simulink model "PropTest"  (R2019b)
settings: Solver=VariableStepAuto  StartTime=0.0  StopTime=40  RelTol=1e-3
values from neighbouring files (symbols this model uses):
  BackProp =     [back_prop.mat]
  ForwProp =     [forward_prop.mat]
undefined symbols (not defined in the file or in its folder): DiscIntNeverNeededParam, motor
libraries: fl_lib x27, nesl_utility x12, sharedutil x3, fl_ps_legacy_lib x3, ee_lib x3, sdl_lib x3, simulink x2
(part 1 of 2)
settings Model: Creator=gonza  LastModifiedBy=gonza

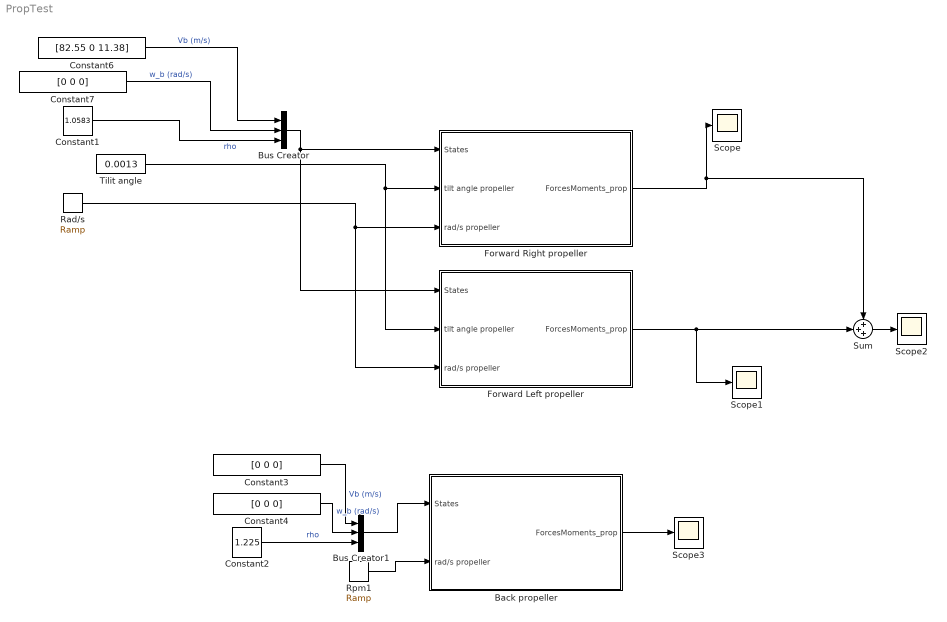
== system PropTest ==
  Back propeller : Subsystem
  Bus Creator : BusCreator  Inputs=3
  Bus Creator1 : BusCreator  Inputs=3
  Constant1 : Constant  Value=1.0583
  Constant2 : Constant  Value=1.225
  Constant3 : Constant  Value=[0 0 0]
  Constant4 : Constant  Value=[0 0 0]
  Constant6 : Constant  Value=[82.55 0 11.38]
  Constant7 : Constant  Value=[0 0 0]
  Forward Left propeller : Subsystem
  Forward Right propeller : Subsystem
  Rad/s : simulink/Sources/Ramp  slope=5  start=5  InitialOutput=10
  Rpm1 : simulink/Sources/Ramp  slope=25  start=5  InitialOutput=0
  Scope{,1..3} (4 alike) : Scope
  Sum : Sum  Inputs=+++
  "Tilit angle " : Constant  Value=0.0013
  wires:
  Bus Creator/1 -> Forward Right propeller/1(States), Forward Left propeller/1(States)
  Constant4/1 -> Bus Creator1/2  "w_b (rad/s)"
  Bus Creator1/1 -> Back propeller/1(States)
  Forward Left propeller/1(ForcesMoments_prop) -> Scope1/1, Sum/2
  Constant1/1 -> Bus Creator/3  "rho"
  Rad/s/1 -> Forward Right propeller/3(rad/s propeller), Forward Left propeller/3(rad/s propeller)
  Forward Right propeller/1(ForcesMoments_prop) -> Scope/1, Sum/1
  Sum/1 -> Scope2/1
  "Tilit angle "/1 -> Forward Right propeller/2(tilt angle propeller), Forward Left propeller/2(tilt angle propeller)
  Constant7/1 -> Bus Creator/2  "w_b (rad/s)"
  Constant2/1 -> Bus Creator1/3  "rho"
  Constant6/1 -> Bus Creator/1  "Vb (m/s)"
  Rpm1/1 -> Back propeller/2(rad/s propeller)
  Constant3/1 -> Bus Creator1/1  "Vb (m/s)"
  Back propeller/1(ForcesMoments_prop) -> Scope3/1

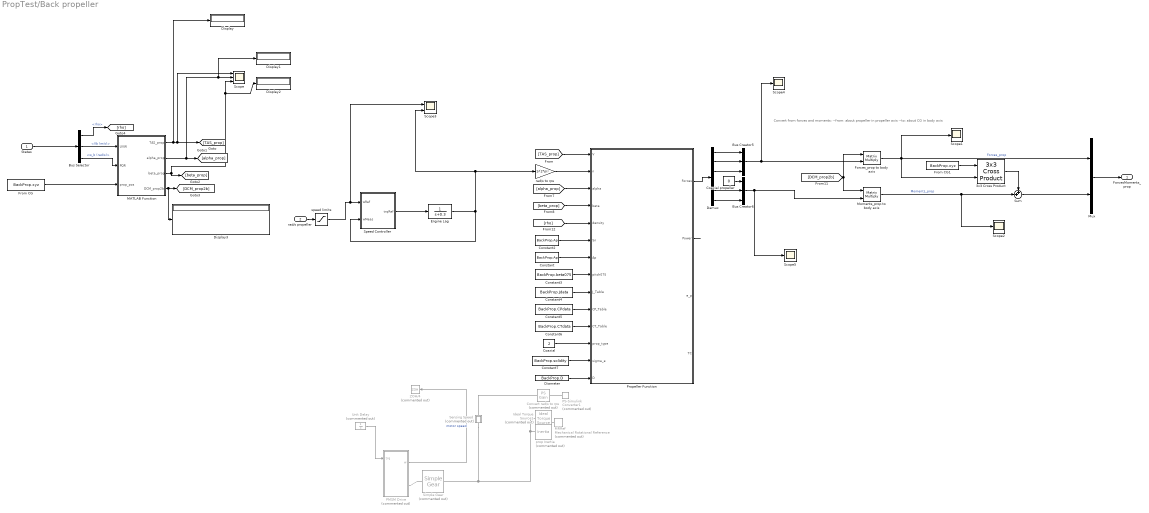
== system PropTest/Back propeller ==
  note: Convert from forces and moments: --from: about propeller in propeller axis --to: about CG in body axis
  States : Inport
  rad/s propeller : Inport  Port=2
  3x3 Cross Product : sharedutil/3x3 Cross Product  aMode=aMode
      settings: SourceProductBaseCode=AE
  Bus Creator5 : BusCreator  Inputs=3
  Bus Creator6 : BusCreator  Inputs=3
  Bus Selector : BusSelector  OutputSignals=rho,Vb (m/s),w_b (rad/s)
  "Coaxial " : Constant  Value=2
  Coaxial propeller : Constant  Value=0
  Constant : Constant  Value=BackProp.Ap
  Constant2 : Constant  Value=BackProp.Ap
  Constant3 : Constant  Value=BackProp.beta075
  Constant4 : Constant  Value=BackProp.Jdata
  Constant5 : Constant  Value=BackProp.CPdata
  Constant6 : Constant  Value=BackProp.CTdata
  Constant7 : Constant  Value=BackProp.solidity
  Convert rad/s to rps : fl_ps_legacy_lib/Legacy Physical Signals/Functions/PS Gain  Commented=on  gain=1/(2*pi)
      settings: SourceProductName=Simscape
  Demux : Demux  Outputs=6
  Diameter : Constant  Value=BackProp.D
  Display{,1..3} (4 alike) : Display
  Engine Lag : TransferFcn  Denominator=[1 0.3]  ContinuousStateAttributes='EngineLag'
  Forces_prop to body axis : Product  Multiplication=Matrix(*)
  From CG : Constant  Value=BackProp.xyz
  From CG1 : Constant  Value=BackProp.xyz
  Ideal Torque Source1 : fl_lib/Mechanical/Mechanical Sources/Ideal Torque Source  Commented=on
  MATLAB Function : MATLAB Function  TreatAsAtomicUnit=on
  MRRef : fl_lib/Mechanical/Rotational Elements/Mechanical Rotational Reference  Commented=on
  Moments_prop to body axis : Product  Multiplication=Matrix(*)
  Mux : Mux  Inputs=2
  PMSM Drive : Subsystem  Tag=PublishSubsystem  Commented=on  VariantControl=Variant1
  PS-Simulink Converter1 : nesl_utility/PS-Simulink Converter  Commented=on  PhysicalDomain=network_engine_domain  SubClassName=ps_output  LeftPortType=input  RightPortType=output  PseudoPeriodic=off  Frequencies=[]  Unit=inherit  AffineConversion=off
  Propeller Function : MATLAB Function  TreatAsAtomicUnit=on
  Scope : Scope  NumInputPorts=3
  Scope{1..2,4..5} (4 alike) : Scope
  Scope3 : Scope  NumInputPorts=2
  Sensing Speed : Subsystem  Commented=on
      mask Display: disp('w')
  Simple Gear : sdl_lib/Gears/Simple Gear  Commented=on  ratio=motor.gear_reduction_forward  rotation_direction=1  friction_model=sdl.enum.gear_efficiencies_load.off  T_noload=0.1 N*m  T_nom=5 N*m  efficiency_nom=0.8  efficiency=0.8  mu_visc=[0, 0] N*m/(rad/s)  w_thr=0.01 rad/s  pwr_thr=0.001 W  enable_faults=simscape.enum.onoff.off  efficiency_fault=0.05  external_fault=simscape.enum.onoff.off  temporal_fault=simscape.enum.onoff.off  fault_time=5 s  fault_angles=pi / 12 rad  report_fault=1  temperature_TLU=[280, 300, 320] K  load_TLU=[1, 5, 10] N*m  efficiency_TLU=[.95, .9, .85]  efficiency_TLU2=[.85, .8, .75; .95, .9, .85; .85, .8, .7]  thermal_mass=50 J/K  T_init=300 K
      settings: SourceProductName=Simscape Driveline
  Speed Controller : Subsystem  mask(P+I motor speed controller){Kp=10, Ki=1, trqMax=20000, ts=0.01}
      mask prompts: Kp "Proportional gain (Nm/(rad/s))"; Ki "Integral gain (Nm/rad)"; trqMax "Maximum torque demand"; ts "Sample time"
      mask help: Inputs wRef and wMeas are the demanded rotor speed and measured rotor speed in rad/s. The controller output is a torque demand in Nm.
  Sum : Sum  Inputs=++|
  Unit Delay : UnitDelay  Commented=on  SampleTime=0.01  HasFrameUpgradeWarning=on
  ZOH/4 : ZeroOrderHold  Commented=on  SampleTime=0.01
  prop Inertia : fl_lib/Mechanical/Rotational Elements/Inertia  Commented=on  inertia="ForwProp.inertia  kg*m^2"  w_specify=on  w_priority=High  w=0 rpm  w_nominal_specify=off  w_nominal_unit=rad/s  w_nominal_value=1  t_specify=off  t_priority=High  t=0 N*m  t_nominal_specify=off  t_nominal_unit=N*m  t_nominal_value=1
  rad/s to rps : Gain  Gain=1/(2*pi)
  speed limits : Saturate  UpperLimit=2000  LowerLimit=-1500
  ForcesMoments_prop : Outport
  wires:
  [rho] -> Propeller Function/5(density)
  MATLAB Function/2(alpha_prop) -> [alpha_prop], Display1/1, Scope/2
  MATLAB Function/3(beta_prop) -> [beta_prop], Scope/3, Display2/1
  Unit Delay/1 -> PMSM Drive/1(trq)
  MATLAB Function/1(TAS_prop) -> Display/1, [TAS_prop], Scope/1
  MATLAB Function/4(DCM_prop2b) -> Display3/1, [DCM_prop2b]
  [TAS_prop] -> Propeller Function/1(V)
  PMSM Drive/1(w) -> ZOH/4/1  "motor speed"
  speed limits/1 -> Scope3/1, Speed Controller/1(wRef)
  From CG/1 -> MATLAB Function/3(prop_pos)
  [alpha_prop] -> Propeller Function/3(alpha)
  rad/s propeller/1 -> speed limits/1
  States/1 -> Bus Selector/1
  Bus Selector/2 -> MATLAB Function/1(UVW)  "<Vb (m/s)>"
  Bus Selector/3 -> MATLAB Function/2(PQR)  "<w_b (rad/s)>"
  Bus Selector/1 -> [rho]  "<rho>"
  Mux/1 -> ForcesMoments_prop/1
  3x3 Cross Product/1 -> Sum/1
  Moments_prop to body axis/1 -> Scope2/1, Sum/2  "Moments_prop"
  Forces_prop to body axis/1 -> Scope1/1, 3x3 Cross Product/2, Mux/1  "Forces_prop"
  [DCM_prop2b] -> Forces_prop to body axis/1, Moments_prop to body axis/1
  From CG1/1 -> 3x3 Cross Product/1
  Bus Creator6/1 -> Scope5/1, Moments_prop to body axis/2
  Sum/1 -> Mux/2
  [beta_prop] -> Propeller Function/4(beta)
  Constant/1 -> Propeller Function/7(Ap)
  Constant2/1 -> Propeller Function/6(Sn)
  Constant3/1 -> Propeller Function/8(pitch075)
  Constant4/1 -> Propeller Function/9(J_Table)
  Constant5/1 -> Propeller Function/10(CP_Table)
  Constant6/1 -> Propeller Function/11(CT_Table)
  Constant7/1 -> Propeller Function/13(sigma_e)
  "Coaxial "/1 -> Propeller Function/12(prop_type)
  Propeller Function/1(Forces) -> Demux/1
  Demux/1 -> Bus Creator5/1
  Demux/6 -> Bus Creator6/3
  Demux/2 -> Bus Creator5/2
  Demux/3 -> Bus Creator5/3
  Demux/5 -> Bus Creator6/2
  Propeller Function/2(Power) -> ?
  Speed Controller/1(trqRef) -> Engine Lag/1
  Engine Lag/1 -> Speed Controller/2(wMeas), Scope3/2, rad/s to rps/1
  Diameter/1 -> Propeller Function/14(D)
  rad/s to rps/1 -> Propeller Function/2(n)
  Coaxial propeller/1 -> Bus Creator6/1
  Bus Creator5/1 -> Scope4/1, Forces_prop to body axis/2
  connections:
  Sensing Speed/LConn1 -- Simple Gear/RConn1 -- prop Inertia/LConn1 -- Ideal Torque Source1/LConn1
  Ideal Torque Source1/RConn2 -- MRRef/LConn1
  Sensing Speed/RConn1 -- Convert rad/s to rps/LConn1
  PS-Simulink Converter1/LConn1 -- Convert rad/s to rps/RConn1
  Simple Gear/LConn1 -- PMSM Drive/RConn1

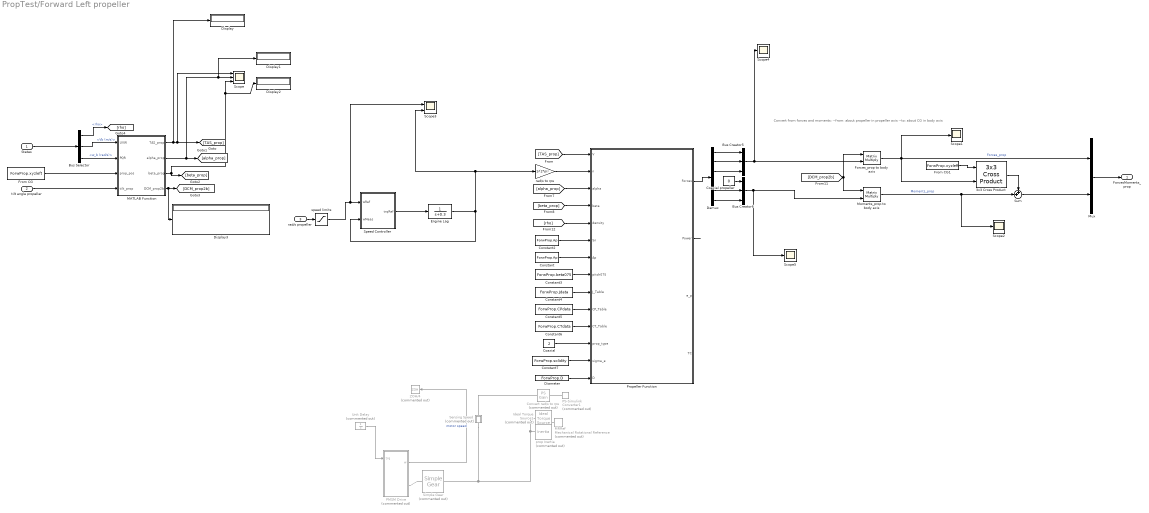
== system PropTest/Forward Left propeller ==
  note: Convert from forces and moments: --from: about propeller in propeller axis --to: about CG in body axis
  States : Inport
  tilt angle propeller : Inport  Port=2
  rad/s propeller : Inport  Port=3
  3x3 Cross Product : sharedutil/3x3 Cross Product  aMode=aMode
      settings: SourceProductBaseCode=AE
  Bus Creator5 : BusCreator  Inputs=3
  Bus Creator6 : BusCreator  Inputs=3
  Bus Selector : BusSelector  OutputSignals=rho,Vb (m/s),w_b (rad/s)
  "Coaxial " : Constant  Value=2
  Coaxial propeller : Constant  Value=0
  Constant : Constant  Value=ForwProp.Ap
  Constant2 : Constant  Value=ForwProp.Ap
  Constant3 : Constant  Value=ForwProp.beta075
  Constant4 : Constant  Value=ForwProp.Jdata
  Constant5 : Constant  Value=ForwProp.CPdata
  Constant6 : Constant  Value=ForwProp.CTdata
  Constant7 : Constant  Value=ForwProp.solidity
  Convert rad/s to rps : fl_ps_legacy_lib/Legacy Physical Signals/Functions/PS Gain  Commented=on  gain=1/(2*pi)
      settings: SourceProductName=Simscape
  Demux : Demux  Outputs=6
  Diameter : Constant  Value=ForwProp.D
  Display{,1..3} (4 alike) : Display
  Engine Lag : TransferFcn  Denominator=[1 0.3]  ContinuousStateAttributes='EngineLag'
  Forces_prop to body axis : Product  Multiplication=Matrix(*)
  From CG : Constant  Value=ForwProp.xyzleft
  From CG1 : Constant  Value=ForwProp.xyzleft
  Ideal Torque Source1 : fl_lib/Mechanical/Mechanical Sources/Ideal Torque Source  Commented=on
  MATLAB Function : MATLAB Function  TreatAsAtomicUnit=on
  MRRef : fl_lib/Mechanical/Rotational Elements/Mechanical Rotational Reference  Commented=on
  Moments_prop to body axis : Product  Multiplication=Matrix(*)
  Mux : Mux  Inputs=2
  PMSM Drive : Subsystem  Tag=PublishSubsystem  Commented=on  VariantControl=Variant1
  PS-Simulink Converter1 : nesl_utility/PS-Simulink Converter  Commented=on  PhysicalDomain=network_engine_domain  SubClassName=ps_output  LeftPortType=input  RightPortType=output  PseudoPeriodic=off  Frequencies=[]  Unit=inherit  AffineConversion=off
  Propeller Function : MATLAB Function  TreatAsAtomicUnit=on
  Scope : Scope  NumInputPorts=3
  Scope{1..2,4..5} (4 alike) : Scope
  Scope3 : Scope  NumInputPorts=2
  Sensing Speed : Subsystem  Commented=on
      mask Display: disp('w')
  Simple Gear : sdl_lib/Gears/Simple Gear  Commented=on  ratio=motor.gear_reduction_forward  rotation_direction=1  friction_model=sdl.enum.gear_efficiencies_load.off  T_noload=0.1 N*m  T_nom=5 N*m  efficiency_nom=0.8  efficiency=0.8  mu_visc=[0, 0] N*m/(rad/s)  w_thr=0.01 rad/s  pwr_thr=0.001 W  enable_faults=simscape.enum.onoff.off  efficiency_fault=0.05  external_fault=simscape.enum.onoff.off  temporal_fault=simscape.enum.onoff.off  fault_time=5 s  fault_angles=pi / 12 rad  report_fault=1  temperature_TLU=[280, 300, 320] K  load_TLU=[1, 5, 10] N*m  efficiency_TLU=[.95, .9, .85]  efficiency_TLU2=[.85, .8, .75; .95, .9, .85; .85, .8, .7]  thermal_mass=50 J/K  T_init=300 K
      settings: SourceProductName=Simscape Driveline
  Speed Controller : Subsystem  mask(P+I motor speed controller){Kp=10, Ki=1, trqMax=20000, ts=0.01}
      mask prompts: Kp "Proportional gain (Nm/(rad/s))"; Ki "Integral gain (Nm/rad)"; trqMax "Maximum torque demand"; ts "Sample time"
      mask help: Inputs wRef and wMeas are the demanded rotor speed and measured rotor speed in rad/s. The controller output is a torque demand in Nm.
  Sum : Sum  Inputs=++|
  Unit Delay : UnitDelay  Commented=on  SampleTime=0.01  HasFrameUpgradeWarning=on
  ZOH/4 : ZeroOrderHold  Commented=on  SampleTime=0.01
  prop Inertia : fl_lib/Mechanical/Rotational Elements/Inertia  Commented=on  inertia="ForwProp.inertia  kg*m^2"  w_specify=on  w_priority=High  w=0 rpm  w_nominal_specify=off  w_nominal_unit=rad/s  w_nominal_value=1  t_specify=off  t_priority=High  t=0 N*m  t_nominal_specify=off  t_nominal_unit=N*m  t_nominal_value=1
  rad/s to rps : Gain  Gain=1/(2*pi)
  speed limits : Saturate  UpperLimit=2000  LowerLimit=-1500
  ForcesMoments_prop : Outport
  wires:
  [rho] -> Propeller Function/5(density)
  MATLAB Function/2(alpha_prop) -> [alpha_prop], Display1/1, Scope/2
  MATLAB Function/3(beta_prop) -> [beta_prop], Scope/3, Display2/1
  Unit Delay/1 -> PMSM Drive/1(trq)
  MATLAB Function/1(TAS_prop) -> Display/1, [TAS_prop], Scope/1
  MATLAB Function/4(DCM_prop2b) -> Display3/1, [DCM_prop2b]
  tilt angle propeller/1 -> MATLAB Function/4(tilt_prop)
  [TAS_prop] -> Propeller Function/1(V)
  PMSM Drive/1(w) -> ZOH/4/1  "motor speed"
  speed limits/1 -> Scope3/1, Speed Controller/1(wRef)
  From CG/1 -> MATLAB Function/3(prop_pos)
  [alpha_prop] -> Propeller Function/3(alpha)
  rad/s propeller/1 -> speed limits/1
  States/1 -> Bus Selector/1
  Bus Selector/2 -> MATLAB Function/1(UVW)  "<Vb (m/s)>"
  Bus Selector/3 -> MATLAB Function/2(PQR)  "<w_b (rad/s)>"
  Bus Selector/1 -> [rho]  "<rho>"
  Mux/1 -> ForcesMoments_prop/1
  3x3 Cross Product/1 -> Sum/1
  Moments_prop to body axis/1 -> Scope2/1, Sum/2  "Moments_prop"
  Forces_prop to body axis/1 -> Scope1/1, 3x3 Cross Product/2, Mux/1  "Forces_prop"
  [DCM_prop2b] -> Forces_prop to body axis/1, Moments_prop to body axis/1
  From CG1/1 -> 3x3 Cross Product/1
  Bus Creator6/1 -> Scope5/1, Moments_prop to body axis/2
  Bus Creator5/1 -> Scope4/1, Forces_prop to body axis/2
  Sum/1 -> Mux/2
  [beta_prop] -> Propeller Function/4(beta)
  Constant/1 -> Propeller Function/7(Ap)
  Constant2/1 -> Propeller Function/6(Sn)
  Constant3/1 -> Propeller Function/8(pitch075)
  Constant4/1 -> Propeller Function/9(J_Table)
  Constant5/1 -> Propeller Function/10(CP_Table)
  Constant6/1 -> Propeller Function/11(CT_Table)
  Constant7/1 -> Propeller Function/13(sigma_e)
  "Coaxial "/1 -> Propeller Function/12(prop_type)
  Propeller Function/1(Forces) -> Demux/1
  Demux/1 -> Bus Creator5/1
  Demux/6 -> Bus Creator6/3
  Demux/2 -> Bus Creator5/2
  Demux/3 -> Bus Creator5/3
  Demux/5 -> Bus Creator6/2
  Propeller Function/2(Power) -> ?
  Speed Controller/1(trqRef) -> Engine Lag/1
  Engine Lag/1 -> Speed Controller/2(wMeas), Scope3/2, rad/s to rps/1
  Diameter/1 -> Propeller Function/14(D)
  rad/s to rps/1 -> Propeller Function/2(n)
  Coaxial propeller/1 -> Bus Creator6/1
  connections:
  Sensing Speed/LConn1 -- Simple Gear/RConn1 -- prop Inertia/LConn1 -- Ideal Torque Source1/LConn1
  Ideal Torque Source1/RConn2 -- MRRef/LConn1
  Sensing Speed/RConn1 -- Convert rad/s to rps/LConn1
  PS-Simulink Converter1/LConn1 -- Convert rad/s to rps/RConn1
  Simple Gear/LConn1 -- PMSM Drive/RConn1

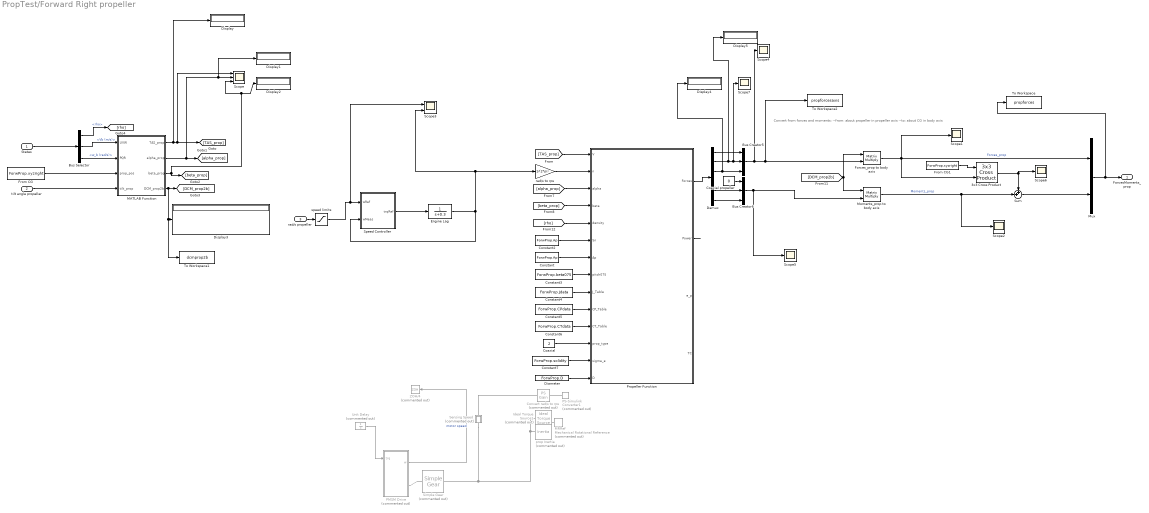
== system PropTest/Forward Right propeller ==
  note: Convert from forces and moments: --from: about propeller in propeller axis --to: about CG in body axis
  States : Inport
  tilt angle propeller : Inport  Port=2
  rad/s propeller : Inport  Port=3
  3x3 Cross Product : sharedutil/3x3 Cross Product  aMode=aMode
      settings: SourceProductBaseCode=AE
  Bus Creator5 : BusCreator  Inputs=3
  Bus Creator6 : BusCreator  Inputs=3
  Bus Selector : BusSelector  OutputSignals=rho,Vb (m/s),w_b (rad/s)
  "Coaxial " : Constant  Value=2
  Coaxial propeller : Constant  Value=0
  Constant : Constant  Value=ForwProp.Ap
  Constant2 : Constant  Value=ForwProp.Ap
  Constant3 : Constant  Value=ForwProp.beta075
  Constant4 : Constant  Value=ForwProp.Jdata
  Constant5 : Constant  Value=ForwProp.CPdata
  Constant6 : Constant  Value=ForwProp.CTdata
  Constant7 : Constant  Value=ForwProp.solidity
  Convert rad/s to rps : fl_ps_legacy_lib/Legacy Physical Signals/Functions/PS Gain  Commented=on  gain=1/(2*pi)
      settings: SourceProductName=Simscape
  Demux : Demux  Outputs=6
  Diameter : Constant  Value=ForwProp.D
  Display{,1..5} (6 alike) : Display
  Engine Lag : TransferFcn  Denominator=[1 0.3]  ContinuousStateAttributes='EngineLag'
  Forces_prop to body axis : Product  Multiplication=Matrix(*)
  From CG : Constant  Value=ForwProp.xyzright
  From CG1 : Constant  Value=ForwProp.xyzright
  Ideal Torque Source1 : fl_lib/Mechanical/Mechanical Sources/Ideal Torque Source  Commented=on
  MATLAB Function : MATLAB Function  TreatAsAtomicUnit=on
  MRRef : fl_lib/Mechanical/Rotational Elements/Mechanical Rotational Reference  Commented=on
  Moments_prop to body axis : Product  Multiplication=Matrix(*)
  Mux : Mux  Inputs=2
  PMSM Drive : Subsystem  Tag=PublishSubsystem  Commented=on  VariantControl=Variant1
  PS-Simulink Converter1 : nesl_utility/PS-Simulink Converter  Commented=on  PhysicalDomain=network_engine_domain  SubClassName=ps_output  LeftPortType=input  RightPortType=output  PseudoPeriodic=off  Frequencies=[]  Unit=inherit  AffineConversion=off
  Propeller Function : MATLAB Function  TreatAsAtomicUnit=on
  Scope : Scope  NumInputPorts=3
  Scope{1..2,4..7} (6 alike) : Scope
  Scope3 : Scope  NumInputPorts=2
  Sensing Speed : Subsystem  Commented=on
      mask Display: disp('w')
  Simple Gear : sdl_lib/Gears/Simple Gear  Commented=on  ratio=motor.gear_reduction_forward  rotation_direction=1  friction_model=sdl.enum.gear_efficiencies_load.off  T_noload=0.1 N*m  T_nom=5 N*m  efficiency_nom=0.8  efficiency=0.8  mu_visc=[0, 0] N*m/(rad/s)  w_thr=0.01 rad/s  pwr_thr=0.001 W  enable_faults=simscape.enum.onoff.off  efficiency_fault=0.05  external_fault=simscape.enum.onoff.off  temporal_fault=simscape.enum.onoff.off  fault_time=5 s  fault_angles=pi / 12 rad  report_fault=1  temperature_TLU=[280, 300, 320] K  load_TLU=[1, 5, 10] N*m  efficiency_TLU=[.95, .9, .85]  efficiency_TLU2=[.85, .8, .75; .95, .9, .85; .85, .8, .7]  thermal_mass=50 J/K  T_init=300 K
      settings: SourceProductName=Simscape Driveline
  Speed Controller : Subsystem  mask(P+I motor speed controller){Kp=10, Ki=1, trqMax=20000, ts=0.01}
      mask prompts: Kp "Proportional gain (Nm/(rad/s))"; Ki "Integral gain (Nm/rad)"; trqMax "Maximum torque demand"; ts "Sample time"
      mask help: Inputs wRef and wMeas are the demanded rotor speed and measured rotor speed in rad/s. The controller output is a torque demand in Nm.
  Sum : Sum  Inputs=++|
  To Workspace : ToWorkspace  VariableName=propforces  SampleTime=-1
  To Workspace1 : ToWorkspace  VariableName=dcmprop2b  SampleTime=-1
  To Workspace2 : ToWorkspace  VariableName=propforcesaxis  SampleTime=-1
  Unit Delay : UnitDelay  Commented=on  SampleTime=0.01  HasFrameUpgradeWarning=on
  ZOH/4 : ZeroOrderHold  Commented=on  SampleTime=0.01
  prop Inertia : fl_lib/Mechanical/Rotational Elements/Inertia  Commented=on  inertia="ForwProp.inertia  kg*m^2"  w_specify=on  w_priority=High  w=0 rpm  w_nominal_specify=off  w_nominal_unit=rad/s  w_nominal_value=1  t_specify=off  t_priority=High  t=0 N*m  t_nominal_specify=off  t_nominal_unit=N*m  t_nominal_value=1
  rad/s to rps : Gain  Gain=1/(2*pi)
  speed limits : Saturate  UpperLimit=2000  LowerLimit=-1500
  ForcesMoments_prop : Outport
  wires:
  [rho] -> Propeller Function/5(density)
  MATLAB Function/2(alpha_prop) -> [alpha_prop], Display1/1, Scope/2
  MATLAB Function/3(beta_prop) -> [beta_prop], Scope/3, Display2/1
  Unit Delay/1 -> PMSM Drive/1(trq)
  MATLAB Function/1(TAS_prop) -> Display/1, [TAS_prop], Scope/1
  MATLAB Function/4(DCM_prop2b) -> To Workspace1/1, Display3/1, [DCM_prop2b]
  tilt angle propeller/1 -> MATLAB Function/4(tilt_prop)
  [TAS_prop] -> Propeller Function/1(V)
  PMSM Drive/1(w) -> ZOH/4/1  "motor speed"
  speed limits/1 -> Scope3/1, Speed Controller/1(wRef)
  From CG/1 -> MATLAB Function/3(prop_pos)
  [alpha_prop] -> Propeller Function/3(alpha)
  rad/s propeller/1 -> speed limits/1
  States/1 -> Bus Selector/1
  Bus Selector/2 -> MATLAB Function/1(UVW)  "<Vb (m/s)>"
  Bus Selector/3 -> MATLAB Function/2(PQR)  "<w_b (rad/s)>"
  Bus Selector/1 -> [rho]  "<rho>"
  Mux/1 -> To Workspace/1, ForcesMoments_prop/1
  3x3 Cross Product/1 -> Scope6/1, Sum/1
  Moments_prop to body axis/1 -> Scope2/1, Sum/2  "Moments_prop"
  Forces_prop to body axis/1 -> Scope1/1, 3x3 Cross Product/2, Mux/1  "Forces_prop"
  [DCM_prop2b] -> Forces_prop to body axis/1, Moments_prop to body axis/1
  From CG1/1 -> 3x3 Cross Product/1
  Bus Creator6/1 -> Scope5/1, Moments_prop to body axis/2
  Bus Creator5/1 -> Scope4/1, To Workspace2/1, Forces_prop to body axis/2
  Sum/1 -> Mux/2
  [beta_prop] -> Propeller Function/4(beta)
  Constant/1 -> Propeller Function/7(Ap)
  Constant2/1 -> Propeller Function/6(Sn)
  Constant3/1 -> Propeller Function/8(pitch075)
  Constant4/1 -> Propeller Function/9(J_Table)
  Constant5/1 -> Propeller Function/10(CP_Table)
  Constant6/1 -> Propeller Function/11(CT_Table)
  Constant7/1 -> Propeller Function/13(sigma_e)
  "Coaxial "/1 -> Propeller Function/12(prop_type)
  Propeller Function/1(Forces) -> Demux/1
  Demux/1 -> Bus Creator5/1
  Demux/6 -> Bus Creator6/3
  Demux/3 -> Display4/1, Bus Creator5/3
  Demux/5 -> Bus Creator6/2
  Propeller Function/2(Power) -> ?
  Speed Controller/1(trqRef) -> Engine Lag/1
  Engine Lag/1 -> Speed Controller/2(wMeas), Scope3/2, rad/s to rps/1
  Diameter/1 -> Propeller Function/14(D)
  rad/s to rps/1 -> Propeller Function/2(n)
  Coaxial propeller/1 -> Bus Creator6/1
  Demux/2 -> Display5/1, Scope7/1, Bus Creator5/2
  connections:
  Sensing Speed/LConn1 -- Simple Gear/RConn1 -- prop Inertia/LConn1 -- Ideal Torque Source1/LConn1
  Ideal Torque Source1/RConn2 -- MRRef/LConn1
  Sensing Speed/RConn1 -- Convert rad/s to rps/LConn1
  PS-Simulink Converter1/LConn1 -- Convert rad/s to rps/RConn1
  Simple Gear/LConn1 -- PMSM Drive/RConn1

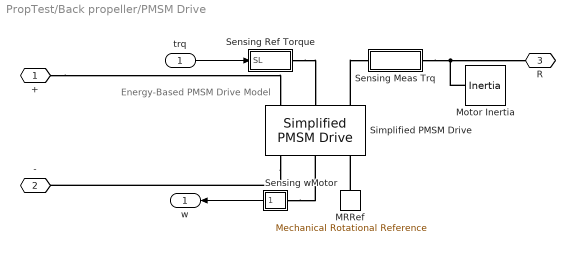
== system PropTest/Back propeller/PMSM Drive ==
  note: Energy-Based
      | PMSM Drive Model
  trq : Inport
  MRRef : fl_lib/Mechanical/Rotational Elements/Mechanical Rotational Reference
  Motor Inertia : fl_lib/Mechanical/Rotational Elements/Inertia  inertia="motor.rotor_inertia  kg*m^2"  w_specify=on  w_priority=High  w=0 rpm  w_nominal_specify=off  w_nominal_unit=rad/s  w_nominal_value=1  t_specify=off  t_priority=High  t=0 N*m  t_nominal_specify=off  t_nominal_unit=N*m  t_nominal_value=1
  Sensing Meas Trq : Subsystem
      mask Display: disp('trqMeas')
  Sensing Ref Torque : Subsystem
      mask Display: disp('trqRef')
  Sensing wMotor : Subsystem
      mask Display: disp('w');
  Simplified PMSM Drive : ee_lib/Electromechanical/Permanent Magnet/Simplified PMSM Drive  torque_speed_param=2  w_t=[0, 3750, 7500, 8000] rpm  T_t=[.09, .08, .07, 0] N*m  torque_max=motor.max_torque N*m  power_max=motor.max_power kW  Tc=0.02 s  losses_param=3  eff=100  w_eff=3750 rpm  T_eff=0.08 N*m  Piron=0 W  Pbase=0 W  w_eff_vec=motor.speed_tab rpm  T_eff_vec=motor.torque_tab N*m  v_eff_vec=[100, 250, 400] V  losses_mat=[1.49, 1.67, 2.21, 3.1; .42, .69, 1.14, 2.03; .06, .24, .78, 1.68; .42, .69, 1.14, 2.03; 1.49, 1.67, 2.21, 3.1] W  efficiency_mat=motor.eff_tab  losses_mat_3D=ones(5, 4, 3) W  efficiency_mat_3D=95 * ones(5, 4, 3)  Res=0 Ohm  J=motor.rotor_inertia kg*m^2  lam=motor.rotor_damping N*m/(rad/s)  speed0=0 rpm  faulted_specify=off  faulted_priority=None  faulted=0  faulted_nominal_specify=off  faulted_nominal_unit=1  faulted_nominal_value=1  alpha=3.93e-3 1/K  Tmeas=25 degC  Tmeas2=125 degC  losses_mat_T2=[1.49, 1.74, 2.49, 3.74; .42, .67, 1.42, 2.67; .06, .31, 1.06, 2.31; .42, .67, 1.42, 2.67; 1.49, 1.74, 2.49, 3.74] W  efficiency_mat_T2=[95, 95, 95, 95; 95, 95, 95, 95; 95, 95, 95, 95; 95, 95, 95, 95; 95, 95, 95, 95]  losses_mat_3D_T2=ones(5, 4, 3) W  efficiency_mat_3D_T2=95 * ones(5, 4, 3)  thermal_mass=100 J/K  initial_temperature=25 degC  fault_condition=1  fault_threshold=0.5
      settings: SourceProductName=Simscape Electrical  SourceProductBaseCode=PS  InternalSimscapePortConfiguration="{\"Bottom\":[],\"Left\":[{\"id\":\"Vp\",\"label\":\"+\",\"type\":\"foundation.electrical.electrical\"},{\"id\":\"Tr\",\"label\":\"Tr\",\"type\":\"input\"},{\"id\":\"R\",\"label\":\"R\",\"type\":\"foundation.mechanical.rotational.rotational\"}],\"Right\":[{\"id\":\"Vm\",\"label\":\"-\",\"type\":\"foundation.electrical.electrical\"},{\"id\":\"Omega\",\"label\":\"w\",\"type\":\"output\"},{\"id\":\"C\",\"label\":\"C\",\"type\":\"foundation.mechanical.rotational.rotational\"}],\"Top\":[]}"
  + : PMIOPort  Side=Left
  - : PMIOPort  Port=2  Side=Left
  R : PMIOPort  Port=3  Side=Right
  w : Outport  VectorParamsAs1DForOutWhenUnconnected=off
  wires:
  trq/1 -> Sensing Ref Torque/1(SL)
  Sensing wMotor/1(SL) -> w/1
  connections:
  Motor Inertia/LConn1 -- Sensing Meas Trq/RConn1 -- R/RConn1
  +/RConn1 -- Simplified PMSM Drive/LConn1
  Sensing wMotor/LConn1 -- Simplified PMSM Drive/RConn2
  Sensing Ref Torque/RConn1 -- Simplified PMSM Drive/LConn2
  MRRef/LConn1 -- Simplified PMSM Drive/RConn3
  Simplified PMSM Drive/RConn1 -- -/RConn1
  Simplified PMSM Drive/LConn3 -- Sensing Meas Trq/LConn1

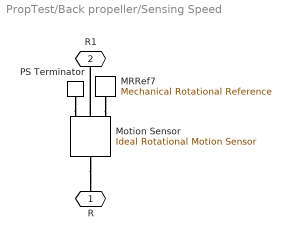
== system PropTest/Back propeller/Sensing Speed ==
  MRRef7 : fl_lib/Mechanical/Rotational Elements/Mechanical Rotational Reference
  Motion Sensor : fl_lib/Mechanical/Mechanical Sensors/Ideal Rotational Motion Sensor  offset=0 rad
  PS Terminator : fl_lib/Physical Signals/Sinks/PS Terminator
      settings: SourceProductName=Simscape
  R : PMIOPort  Side=Left
  R1 : PMIOPort  Port=2  Side=Right
  connections:
  Motion Sensor/LConn1 -- R/RConn1
  MRRef7/LConn1 -- Motion Sensor/RConn1
  Motion Sensor/RConn2 -- R1/RConn1
  PS Terminator/LConn1 -- Motion Sensor/RConn3

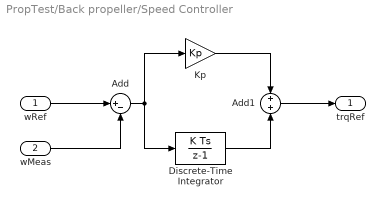
== system PropTest/Back propeller/Speed Controller ==
  wRef : Inport
  wMeas : Inport  Port=2
  Add : Sum  Inputs=|+-
  Add1 : Sum
  Discrete-Time Integrator : DiscreteIntegrator  gainval=Ki  SampleTime=ts  LimitOutput=on  UpperSaturationLimit=trqMax  LowerSaturationLimit=-trqMax  ICPrevOutput=DiscIntNeverNeededParam  ICPrevScaledInput=DiscIntNeverNeededParam
  Kp : Gain  Gain=Kp
  trqRef : Outport  VectorParamsAs1DForOutWhenUnconnected=off
  wires:
  wRef/1 -> Add/1
  Kp/1 -> Add1/1
  Discrete-Time Integrator/1 -> Add1/2
  wMeas/1 -> Add/2
  Add1/1 -> trqRef/1
  Add/1 -> Kp/1, Discrete-Time Integrator/1

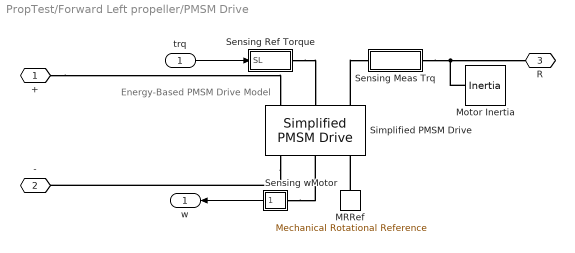
== system PropTest/Forward Left propeller/PMSM Drive ==
  note: Energy-Based
      | PMSM Drive Model
  trq : Inport
  MRRef : fl_lib/Mechanical/Rotational Elements/Mechanical Rotational Reference
  Motor Inertia : fl_lib/Mechanical/Rotational Elements/Inertia  inertia="motor.rotor_inertia  kg*m^2"  w_specify=on  w_priority=High  w=0 rpm  w_nominal_specify=off  w_nominal_unit=rad/s  w_nominal_value=1  t_specify=off  t_priority=High  t=0 N*m  t_nominal_specify=off  t_nominal_unit=N*m  t_nominal_value=1
  Sensing Meas Trq : Subsystem
      mask Display: disp('trqMeas')
  Sensing Ref Torque : Subsystem
      mask Display: disp('trqRef')
  Sensing wMotor : Subsystem
      mask Display: disp('w');
  Simplified PMSM Drive : ee_lib/Electromechanical/Permanent Magnet/Simplified PMSM Drive  torque_speed_param=2  w_t=[0, 3750, 7500, 8000] rpm  T_t=[.09, .08, .07, 0] N*m  torque_max=motor.max_torque N*m  power_max=motor.max_power kW  Tc=0.02 s  losses_param=3  eff=100  w_eff=3750 rpm  T_eff=0.08 N*m  Piron=0 W  Pbase=0 W  w_eff_vec=motor.speed_tab rpm  T_eff_vec=motor.torque_tab N*m  v_eff_vec=[100, 250, 400] V  losses_mat=[1.49, 1.67, 2.21, 3.1; .42, .69, 1.14, 2.03; .06, .24, .78, 1.68; .42, .69, 1.14, 2.03; 1.49, 1.67, 2.21, 3.1] W  efficiency_mat=motor.eff_tab  losses_mat_3D=ones(5, 4, 3) W  efficiency_mat_3D=95 * ones(5, 4, 3)  Res=0 Ohm  J=motor.rotor_inertia kg*m^2  lam=motor.rotor_damping N*m/(rad/s)  speed0=0 rpm  faulted_specify=off  faulted_priority=None  faulted=0  faulted_nominal_specify=off  faulted_nominal_unit=1  faulted_nominal_value=1  alpha=3.93e-3 1/K  Tmeas=25 degC  Tmeas2=125 degC  losses_mat_T2=[1.49, 1.74, 2.49, 3.74; .42, .67, 1.42, 2.67; .06, .31, 1.06, 2.31; .42, .67, 1.42, 2.67; 1.49, 1.74, 2.49, 3.74] W  efficiency_mat_T2=[95, 95, 95, 95; 95, 95, 95, 95; 95, 95, 95, 95; 95, 95, 95, 95; 95, 95, 95, 95]  losses_mat_3D_T2=ones(5, 4, 3) W  efficiency_mat_3D_T2=95 * ones(5, 4, 3)  thermal_mass=100 J/K  initial_temperature=25 degC  fault_condition=1  fault_threshold=0.5
      settings: SourceProductName=Simscape Electrical  SourceProductBaseCode=PS  InternalSimscapePortConfiguration="{\"Bottom\":[],\"Left\":[{\"id\":\"Vp\",\"label\":\"+\",\"type\":\"foundation.electrical.electrical\"},{\"id\":\"Tr\",\"label\":\"Tr\",\"type\":\"input\"},{\"id\":\"R\",\"label\":\"R\",\"type\":\"foundation.mechanical.rotational.rotational\"}],\"Right\":[{\"id\":\"Vm\",\"label\":\"-\",\"type\":\"foundation.electrical.electrical\"},{\"id\":\"Omega\",\"label\":\"w\",\"type\":\"output\"},{\"id\":\"C\",\"label\":\"C\",\"type\":\"foundation.mechanical.rotational.rotational\"}],\"Top\":[]}"
  + : PMIOPort  Side=Left
  - : PMIOPort  Port=2  Side=Left
  R : PMIOPort  Port=3  Side=Right
  w : Outport  VectorParamsAs1DForOutWhenUnconnected=off
  wires:
  trq/1 -> Sensing Ref Torque/1(SL)
  Sensing wMotor/1(SL) -> w/1
  connections:
  Motor Inertia/LConn1 -- Sensing Meas Trq/RConn1 -- R/RConn1
  +/RConn1 -- Simplified PMSM Drive/LConn1
  Sensing wMotor/LConn1 -- Simplified PMSM Drive/RConn2
  Sensing Ref Torque/RConn1 -- Simplified PMSM Drive/LConn2
  MRRef/LConn1 -- Simplified PMSM Drive/RConn3
  Simplified PMSM Drive/RConn1 -- -/RConn1
  Simplified PMSM Drive/LConn3 -- Sensing Meas Trq/LConn1

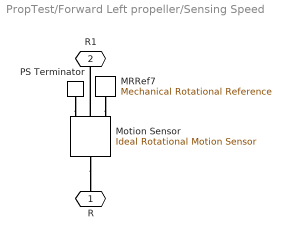
== system PropTest/Forward Left propeller/Sensing Speed ==
  MRRef7 : fl_lib/Mechanical/Rotational Elements/Mechanical Rotational Reference
  Motion Sensor : fl_lib/Mechanical/Mechanical Sensors/Ideal Rotational Motion Sensor  offset=0 rad
  PS Terminator : fl_lib/Physical Signals/Sinks/PS Terminator
      settings: SourceProductName=Simscape
  R : PMIOPort  Side=Left
  R1 : PMIOPort  Port=2  Side=Right
  connections:
  Motion Sensor/LConn1 -- R/RConn1
  MRRef7/LConn1 -- Motion Sensor/RConn1
  Motion Sensor/RConn2 -- R1/RConn1
  PS Terminator/LConn1 -- Motion Sensor/RConn3

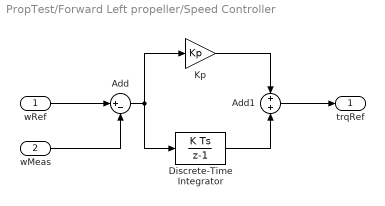
== system PropTest/Forward Left propeller/Speed Controller ==
  wRef : Inport
  wMeas : Inport  Port=2
  Add : Sum  Inputs=|+-
  Add1 : Sum
  Discrete-Time Integrator : DiscreteIntegrator  gainval=Ki  SampleTime=ts  LimitOutput=on  UpperSaturationLimit=trqMax  LowerSaturationLimit=-trqMax  ICPrevOutput=DiscIntNeverNeededParam  ICPrevScaledInput=DiscIntNeverNeededParam
  Kp : Gain  Gain=Kp
  trqRef : Outport  VectorParamsAs1DForOutWhenUnconnected=off
  wires:
  wRef/1 -> Add/1
  Kp/1 -> Add1/1
  Discrete-Time Integrator/1 -> Add1/2
  wMeas/1 -> Add/2
  Add1/1 -> trqRef/1
  Add/1 -> Kp/1, Discrete-Time Integrator/1

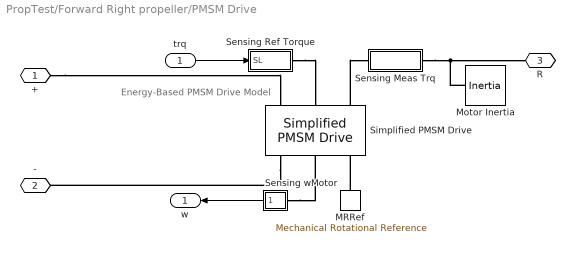
== system PropTest/Forward Right propeller/PMSM Drive ==
  note: Energy-Based
      | PMSM Drive Model
  trq : Inport
  MRRef : fl_lib/Mechanical/Rotational Elements/Mechanical Rotational Reference
  Motor Inertia : fl_lib/Mechanical/Rotational Elements/Inertia  inertia="motor.rotor_inertia  kg*m^2"  w_specify=on  w_priority=High  w=0 rpm  w_nominal_specify=off  w_nominal_unit=rad/s  w_nominal_value=1  t_specify=off  t_priority=High  t=0 N*m  t_nominal_specify=off  t_nominal_unit=N*m  t_nominal_value=1
  Sensing Meas Trq : Subsystem
      mask Display: disp('trqMeas')
  Sensing Ref Torque : Subsystem
      mask Display: disp('trqRef')
  Sensing wMotor : Subsystem
      mask Display: disp('w');
  Simplified PMSM Drive : ee_lib/Electromechanical/Permanent Magnet/Simplified PMSM Drive  torque_speed_param=2  w_t=[0, 3750, 7500, 8000] rpm  T_t=[.09, .08, .07, 0] N*m  torque_max=motor.max_torque N*m  power_max=motor.max_power kW  Tc=0.02 s  losses_param=3  eff=100  w_eff=3750 rpm  T_eff=0.08 N*m  Piron=0 W  Pbase=0 W  w_eff_vec=motor.speed_tab rpm  T_eff_vec=motor.torque_tab N*m  v_eff_vec=[100, 250, 400] V  losses_mat=[1.49, 1.67, 2.21, 3.1; .42, .69, 1.14, 2.03; .06, .24, .78, 1.68; .42, .69, 1.14, 2.03; 1.49, 1.67, 2.21, 3.1] W  efficiency_mat=motor.eff_tab  losses_mat_3D=ones(5, 4, 3) W  efficiency_mat_3D=95 * ones(5, 4, 3)  Res=0 Ohm  J=motor.rotor_inertia kg*m^2  lam=motor.rotor_damping N*m/(rad/s)  speed0=0 rpm  faulted_specify=off  faulted_priority=None  faulted=0  faulted_nominal_specify=off  faulted_nominal_unit=1  faulted_nominal_value=1  alpha=3.93e-3 1/K  Tmeas=25 degC  Tmeas2=125 degC  losses_mat_T2=[1.49, 1.74, 2.49, 3.74; .42, .67, 1.42, 2.67; .06, .31, 1.06, 2.31; .42, .67, 1.42, 2.67; 1.49, 1.74, 2.49, 3.74] W  efficiency_mat_T2=[95, 95, 95, 95; 95, 95, 95, 95; 95, 95, 95, 95; 95, 95, 95, 95; 95, 95, 95, 95]  losses_mat_3D_T2=ones(5, 4, 3) W  efficiency_mat_3D_T2=95 * ones(5, 4, 3)  thermal_mass=100 J/K  initial_temperature=25 degC  fault_condition=1  fault_threshold=0.5
      settings: SourceProductName=Simscape Electrical  SourceProductBaseCode=PS  InternalSimscapePortConfiguration="{\"Bottom\":[],\"Left\":[{\"id\":\"Vp\",\"label\":\"+\",\"type\":\"foundation.electrical.electrical\"},{\"id\":\"Tr\",\"label\":\"Tr\",\"type\":\"input\"},{\"id\":\"R\",\"label\":\"R\",\"type\":\"foundation.mechanical.rotational.rotational\"}],\"Right\":[{\"id\":\"Vm\",\"label\":\"-\",\"type\":\"foundation.electrical.electrical\"},{\"id\":\"Omega\",\"label\":\"w\",\"type\":\"output\"},{\"id\":\"C\",\"label\":\"C\",\"type\":\"foundation.mechanical.rotational.rotational\"}],\"Top\":[]}"
  + : PMIOPort  Side=Left
  - : PMIOPort  Port=2  Side=Left
  R : PMIOPort  Port=3  Side=Right
  w : Outport  VectorParamsAs1DForOutWhenUnconnected=off
  wires:
  trq/1 -> Sensing Ref Torque/1(SL)
  Sensing wMotor/1(SL) -> w/1
  connections:
  Motor Inertia/LConn1 -- Sensing Meas Trq/RConn1 -- R/RConn1
  +/RConn1 -- Simplified PMSM Drive/LConn1
  Sensing wMotor/LConn1 -- Simplified PMSM Drive/RConn2
  Sensing Ref Torque/RConn1 -- Simplified PMSM Drive/LConn2
  MRRef/LConn1 -- Simplified PMSM Drive/RConn3
  Simplified PMSM Drive/RConn1 -- -/RConn1
  Simplified PMSM Drive/LConn3 -- Sensing Meas Trq/LConn1

== system PropTest/Forward Right propeller/Sensing Speed ==
  MRRef7 : fl_lib/Mechanical/Rotational Elements/Mechanical Rotational Reference
  Motion Sensor : fl_lib/Mechanical/Mechanical Sensors/Ideal Rotational Motion Sensor  offset=0 rad
  PS Terminator : fl_lib/Physical Signals/Sinks/PS Terminator
      settings: SourceProductName=Simscape
  R : PMIOPort  Side=Left
  R1 : PMIOPort  Port=2  Side=Right
  connections:
  Motion Sensor/LConn1 -- R/RConn1
  MRRef7/LConn1 -- Motion Sensor/RConn1
  Motion Sensor/RConn2 -- R1/RConn1
  PS Terminator/LConn1 -- Motion Sensor/RConn3

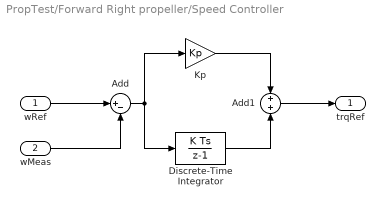
== system PropTest/Forward Right propeller/Speed Controller ==
  wRef : Inport
  wMeas : Inport  Port=2
  Add : Sum  Inputs=|+-
  Add1 : Sum
  Discrete-Time Integrator : DiscreteIntegrator  gainval=Ki  SampleTime=ts  LimitOutput=on  UpperSaturationLimit=trqMax  LowerSaturationLimit=-trqMax  ICPrevOutput=DiscIntNeverNeededParam  ICPrevScaledInput=DiscIntNeverNeededParam
  Kp : Gain  Gain=Kp
  trqRef : Outport  VectorParamsAs1DForOutWhenUnconnected=off
  wires:
  wRef/1 -> Add/1
  Kp/1 -> Add1/1
  Discrete-Time Integrator/1 -> Add1/2
  wMeas/1 -> Add/2
  Add1/1 -> trqRef/1
  Add/1 -> Kp/1, Discrete-Time Integrator/1

== system PropTest/Back propeller/PMSM Drive/Sensing Meas Trq ==
  Ideal Torque Sensor : fl_lib/Mechanical/Mechanical Sensors/Ideal Torque Sensor
  PS-Simulink Converter2 : nesl_utility/PS-Simulink Converter  PhysicalDomain=network_engine_domain  SubClassName=ps_output  LeftPortType=input  RightPortType=output  PseudoPeriodic=off  Frequencies=[]  Unit=N*m  AffineConversion=off
  R : PMIOPort  Side=Left
  C : PMIOPort  Port=2  Side=Right
  tag scope: trqMotor=global
  wires:
  PS-Simulink Converter2/1 -> [trqMotor]
  connections:
  C/RConn1 -- Ideal Torque Sensor/RConn1
  R/RConn1 -- Ideal Torque Sensor/LConn1
  Ideal Torque Sensor/RConn2 -- PS-Simulink Converter2/LConn1

== system PropTest/Back propeller/PMSM Drive/Sensing Ref Torque ==
  SL : Inport
  Simulink-PS G1 : nesl_utility/Simulink-PS Converter  PhysicalDomain=network_engine_domain  SubClassName=ps_input  LeftPortType=input  RightPortType=output  PseudoPeriodic=off  Frequencies=[]  NoiseDistribution=none  NoiseParameters=[]  Unit=1  AffineConversion=off  FilteringAndDerivatives=zero  SimscapeFilterOrder=1  InputFilterTimeConstant=1e-6  UdotUserProvided=1
  PS : PMIOPort  Side=Right
  tag scope: trq_demand=global
  wires:
  SL/1 -> [trq_demand], Simulink-PS G1/1
  connections:
  Simulink-PS G1/RConn1 -- PS/RConn1

== system PropTest/Back propeller/PMSM Drive/Sensing wMotor ==
  PS-Simulink Converter : nesl_utility/PS-Simulink Converter  PhysicalDomain=network_engine_domain  SubClassName=ps_output  LeftPortType=input  RightPortType=output  PseudoPeriodic=off  Frequencies=[]  Unit=rad/s  AffineConversion=off
  PS : PMIOPort  Side=Left
  SL : Outport  VectorParamsAs1DForOutWhenUnconnected=off
  tag scope: wMotor=global
  wires:
  PS-Simulink Converter/1 -> SL/1, [wMotor]
  connections:
  PS/RConn1 -- PS-Simulink Converter/LConn1

== system PropTest/Forward Left propeller/PMSM Drive/Sensing Meas Trq ==
  Ideal Torque Sensor : fl_lib/Mechanical/Mechanical Sensors/Ideal Torque Sensor
  PS-Simulink Converter2 : nesl_utility/PS-Simulink Converter  PhysicalDomain=network_engine_domain  SubClassName=ps_output  LeftPortType=input  RightPortType=output  PseudoPeriodic=off  Frequencies=[]  Unit=N*m  AffineConversion=off
  R : PMIOPort  Side=Left
  C : PMIOPort  Port=2  Side=Right
  tag scope: trqMotor=global
  wires:
  PS-Simulink Converter2/1 -> [trqMotor]
  connections:
  C/RConn1 -- Ideal Torque Sensor/RConn1
  R/RConn1 -- Ideal Torque Sensor/LConn1
  Ideal Torque Sensor/RConn2 -- PS-Simulink Converter2/LConn1

== system PropTest/Forward Left propeller/PMSM Drive/Sensing Ref Torque ==
  SL : Inport
  Simulink-PS G1 : nesl_utility/Simulink-PS Converter  PhysicalDomain=network_engine_domain  SubClassName=ps_input  LeftPortType=input  RightPortType=output  PseudoPeriodic=off  Frequencies=[]  NoiseDistribution=none  NoiseParameters=[]  Unit=1  AffineConversion=off  FilteringAndDerivatives=zero  SimscapeFilterOrder=1  InputFilterTimeConstant=1e-6  UdotUserProvided=1
  PS : PMIOPort  Side=Right
  tag scope: trq_demand=global
  wires:
  SL/1 -> [trq_demand], Simulink-PS G1/1
  connections:
  Simulink-PS G1/RConn1 -- PS/RConn1

== system PropTest/Forward Left propeller/PMSM Drive/Sensing wMotor ==
  PS-Simulink Converter : nesl_utility/PS-Simulink Converter  PhysicalDomain=network_engine_domain  SubClassName=ps_output  LeftPortType=input  RightPortType=output  PseudoPeriodic=off  Frequencies=[]  Unit=rad/s  AffineConversion=off
  PS : PMIOPort  Side=Left
  SL : Outport  VectorParamsAs1DForOutWhenUnconnected=off
  tag scope: wMotor=global
  wires:
  PS-Simulink Converter/1 -> SL/1, [wMotor]
  connections:
  PS/RConn1 -- PS-Simulink Converter/LConn1

== system PropTest/Forward Right propeller/PMSM Drive/Sensing Meas Trq ==
  Ideal Torque Sensor : fl_lib/Mechanical/Mechanical Sensors/Ideal Torque Sensor
  PS-Simulink Converter2 : nesl_utility/PS-Simulink Converter  PhysicalDomain=network_engine_domain  SubClassName=ps_output  LeftPortType=input  RightPortType=output  PseudoPeriodic=off  Frequencies=[]  Unit=N*m  AffineConversion=off
  R : PMIOPort  Side=Left
  C : PMIOPort  Port=2  Side=Right
  tag scope: trqMotor=global
  wires:
  PS-Simulink Converter2/1 -> [trqMotor]
  connections:
  C/RConn1 -- Ideal Torque Sensor/RConn1
  R/RConn1 -- Ideal Torque Sensor/LConn1
  Ideal Torque Sensor/RConn2 -- PS-Simulink Converter2/LConn1

== system PropTest/Forward Right propeller/PMSM Drive/Sensing Ref Torque ==
  SL : Inport
  Simulink-PS G1 : nesl_utility/Simulink-PS Converter  PhysicalDomain=network_engine_domain  SubClassName=ps_input  LeftPortType=input  RightPortType=output  PseudoPeriodic=off  Frequencies=[]  NoiseDistribution=none  NoiseParameters=[]  Unit=1  AffineConversion=off  FilteringAndDerivatives=zero  SimscapeFilterOrder=1  InputFilterTimeConstant=1e-6  UdotUserProvided=1
  PS : PMIOPort  Side=Right
  tag scope: trq_demand=global
  wires:
  SL/1 -> [trq_demand], Simulink-PS G1/1
  connections:
  Simulink-PS G1/RConn1 -- PS/RConn1

== system PropTest/Forward Right propeller/PMSM Drive/Sensing wMotor ==
  PS-Simulink Converter : nesl_utility/PS-Simulink Converter  PhysicalDomain=network_engine_domain  SubClassName=ps_output  LeftPortType=input  RightPortType=output  PseudoPeriodic=off  Frequencies=[]  Unit=rad/s  AffineConversion=off
  PS : PMIOPort  Side=Left
  SL : Outport  VectorParamsAs1DForOutWhenUnconnected=off
  tag scope: wMotor=global
  wires:
  PS-Simulink Converter/1 -> SL/1, [wMotor]
  connections:
  PS/RConn1 -- PS-Simulink Converter/LConn1

== matlab function PropTest/Back propeller/Propeller Function ==
  data: V input; Forces output; n input; alpha input; beta input; density input; Sn input; Ap input; pitch075 input; J_Table input; CP_Table input; CT_Table input; prop_type input; sigma_e input; Power output; e_p output; TC output; D input
function [Forces,Power,e_p,TC] = prop_model(V,n, alpha,beta,density,Sn,Ap,pitch075,...
                           J_Table,CP_Table,CT_Table,prop_type,sigma_e,D)
%prop_model: Propeller power and forces calculation in the spinner axis. 
% Method based on strip theory which was applicable to small or moderate
% inclination angles (approx. <20deg). The method also calculates the prop
% downwash caused by the slipstream.
% V:        Airspeed (m/s)
% n:        Rotor speed (rps) (<0 if prop rotates clockwise)
% alpha: 	Rotor angle of attack (rad)
% beta:     Rotor sideslip (rad)
% density:  Air density
%
% Sn:       Nacelle area
% Ap        prop disk area
% pitch075:    Prop pitch angle referred to zero-lift line of section 0.75R (deg)
% J_Table:  Table of advance ratio
% CP_Table: Table of CP
% CT_Table: Table of CT
% prop_type: 1 single prop, 2 coaxial prop
% sigma_e:  Propeller solidity

if n ~= 0
    % advance ratio
    J = V /(abs(n)* D);
else
    J = 0;
end
% corrected advance ratio
% ESDU86017
Jeff = J * (1 - 0.255*Sn/Ap);

% propeller CP
CP = interp1(J_Table,CP_Table,Jeff,'linear','extrap');      
% propeller CT
CT = interp1(J_Table,CT_Table,Jeff,'linear','extrap');

if J ~= 0
    % ESDU 89047 
    Tc = CT * 8/(pi * J^2);
    kb = tan(pi/180*(pitch075 - 5))/(sigma_e * cos(pi/180*(pitch075 - 5)));
    if prop_type == 1
        CZ_alpha = -((4.25 * sigma_e)/(1 + 2 * sigma_e)) * sin(pi/180*(pitch075 + 3))*...
            (1 + ((3 * Tc/8)/sqrt(1 + (2*Tc/3))));  
        Cn_CZ = -(0.321/(sigma_e + tan(pi/180*(pitch075 + 5)))) * (1 + ((Tc * kb/3)...
            /(1 + (3 * Tc * sqrt(kb)/4))));
        CZ_alpha = CZ_alpha * (CT/Tc); 
        Cn_alpha = Cn_CZ * CZ_alpha;
    else
        CZ_alpha = -((3.86 * sigma_e)/(1 + sigma_e)) * sin(pi/180*(pitch075 + 9))*...
            (1 + ((3 * Tc/8)/sqrt(1 + (2*Tc/3))));
        CZ_alpha = CZ_alpha * (CT/Tc);   
        Cn_alpha = 0;
    end
else
    Tc=0;
    
    CZ_alpha =0;
    Cn_alpha =0;
end
Forces = zeros(6,1); 

%CT>0
% correction based on ESDU86017 for nacelle effect
Forces(1) = density*n^2*D^4*CT*(1 - 0.255*Sn/Ap);
% CY_beta sign of n (<0 if clockwise) 
Forces(2) = -sign(n)*density*n^2*D^4*CZ_alpha*beta;
% CZ_apha < 0 
Forces(3) = density*n^2*D^4*CZ_alpha*alpha;
Forces(4) = density*n^2*D^5*CP/(2*pi);
% Cm_beta sign of n (<0 if clockwise) 
Forces(5) = sign(n)*density*n^2*D^5*Cn_alpha*beta;
% Cn_alpha - sign of n (>0 if clockwise) 
Forces(6) = - sign(n)*density*n^2*D^5*Cn_alpha*beta;
       
Power = density*n^2*D^5*CP;

% Downwash caused by propeller slipstream based on LabanOn-line Aircraft
% Aerodynamic Model Identification. PhD thesis, Proefschrift Technische
% Universiteit Delft, 1994.
e_p = (Forces(1)*sin(alpha)-Forces(3)*cos(alpha))/(density*V^2*Ap);
TC = Tc*pi/8;

if V>40
    Forces = zeros(6,1); 
end
    
   
end

== matlab function PropTest/Forward Left propeller/MATLAB Function ==
  data: UVW input; TAS_prop output; PQR input; prop_pos input; tilt_prop input; alpha_prop output; beta_prop output; DCM_prop2b output
function [TAS_prop,alpha_prop,beta_prop,DCM_prop2b] = fcn(UVW,PQR,prop_pos,tilt_prop)
%Initialize vectors
UVW = [UVW(1) UVW(2) UVW(3)];
PQR = [PQR(1) PQR(2) PQR(3)];
prop_pos = [prop_pos(1) prop_pos(2) prop_pos(3)];

%UVW calculation v = v0 + w^r (rigid body) 
UVW_prop = UVW + cross(PQR,prop_pos);

%outputs
TAS_prop = norm(UVW_prop);


if TAS_prop<10
    alpha_prop=0;
    beta_prop=0;
else
    alpha_prop = tilt_prop + atan(UVW_prop(3)/UVW_prop(1));
    beta_prop = asin(UVW_prop(2)/TAS_prop);
end

DCM_prop2b = [cos(tilt_prop) 0 sin(tilt_prop);
        0 1 0;
        -sin(tilt_prop) 0 cos(tilt_prop)];
    
end

== matlab function PropTest/Forward Right propeller/MATLAB Function ==
  data: UVW input; TAS_prop output; PQR input; prop_pos input; tilt_prop input; alpha_prop output; beta_prop output; DCM_prop2b output
function [TAS_prop,alpha_prop,beta_prop,DCM_prop2b] = fcn(UVW,PQR,prop_pos,tilt_prop)
%Initialize vectors
UVW = [UVW(1) UVW(2) UVW(3)];
PQR = [PQR(1) PQR(2) PQR(3)];
prop_pos = [prop_pos(1) prop_pos(2) prop_pos(3)];

%UVW calculation v = v0 + w^r (rigid body) 
UVW_prop = UVW + cross(PQR,prop_pos);

%outputs
TAS_prop = norm(UVW_prop);


if TAS_prop<10
    alpha_prop=0;
    beta_prop=0;
else
    alpha_prop = tilt_prop + atan(UVW_prop(3)/UVW_prop(1));
    beta_prop = asin(UVW_prop(2)/TAS_prop);
end

DCM_prop2b = [cos(tilt_prop) 0 sin(tilt_prop);
        0 1 0;
        -sin(tilt_prop) 0 cos(tilt_prop)];
    
end

== matlab function PropTest/Forward Left propeller/Propeller Function ==
  data: V input; Forces output; n input; alpha input; beta input; density input; Sn input; Ap input; pitch075 input; J_Table input; CP_Table input; CT_Table input; prop_type input; sigma_e input; Power output; e_p output; TC output; D input
function [Forces,Power,e_p,TC] = prop_model(V,n, alpha,beta,density,Sn,Ap,pitch075,...
                           J_Table,CP_Table,CT_Table,prop_type,sigma_e,D)
%prop_model: Propeller power and forces calculation in the spinner axis. 
% Method based on strip theory which was applicable to small or moderate
% inclination angles (approx. <20deg). The method also calculates the prop
% downwash caused by the slipstream.
% V:        Airspeed (m/s)
% n:        Rotor speed (rps) (<0 if prop rotates clockwise)
% alpha: 	Rotor angle of attack (rad)
% beta:     Rotor sideslip (rad)
% density:  Air density
%
% Sn:       Nacelle area
% Ap        prop disk area
% pitch075:    Prop pitch angle referred to zero-lift line of section 0.75R (deg)
% J_Table:  Table of advance ratio
% CP_Table: Table of CP
% CT_Table: Table of CT
% prop_type: 1 single prop, 2 coaxial prop
% sigma_e:  Propeller solidity

if n ~= 0
    % advance ratio
    J = V /(abs(n)* D);
else
    J = 0;
end
% corrected advance ratio
% ESDU86017
Jeff = J * (1 - 0.255*Sn/Ap);

% propeller CP
CP = interp1(J_Table,CP_Table,Jeff,'linear','extrap');      
% propeller CT
CT = interp1(J_Table,CT_Table,Jeff,'linear','extrap');

if J ~= 0
    % ESDU 89047 
    Tc = CT * 8/(pi * J^2);
    kb = tan(pi/180*(pitch075 - 5))/(sigma_e * cos(pi/180*(pitch075 - 5)));
    if prop_type == 1
        CZ_alpha = -((4.25 * sigma_e)/(1 + 2 * sigma_e)) * sin(pi/180*(pitch075 + 3))*...
            (1 + ((3 * Tc/8)/sqrt(1 + (2*Tc/3))));  
        Cn_CZ = -(0.321/(sigma_e + tan(pi/180*(pitch075 + 5)))) * (1 + ((Tc * kb/3)...
            /(1 + (3 * Tc * sqrt(kb)/4))));
        CZ_alpha = CZ_alpha * (CT/Tc); 
        Cn_alpha = Cn_CZ * CZ_alpha;
    else
        CZ_alpha = -((3.86 * sigma_e)/(1 + sigma_e)) * sin(pi/180*(pitch075 + 9))*...
            (1 + ((3 * Tc/8)/sqrt(1 + (2*Tc/3))));
        CZ_alpha = CZ_alpha * (CT/Tc);   
        Cn_alpha = 0;
    end
else
    Tc=0;
    
    CZ_alpha =0;
    Cn_alpha =0;
end
Forces = zeros(6,1); 

%CT>0
% correction based on ESDU86017 for nacelle effect
Forces(1) = density*n^2*D^4*CT*(1 - 0.255*Sn/Ap);
% CY_beta sign of n (<0 if clockwise) 
Forces(2) = -sign(n)*density*n^2*D^4*CZ_alpha*beta;
% CZ_apha < 0 
Forces(3) = density*n^2*D^4*CZ_alpha*alpha;
Forces(4) = density*n^2*D^5*CP/(2*pi);
% Cm_beta sign of n (<0 if clockwise) 
Forces(5) = sign(n)*density*n^2*D^5*Cn_alpha*beta;
% Cn_alpha - sign of n (>0 if clockwise) 
Forces(6) = - sign(n)*density*n^2*D^5*Cn_alpha*beta;
       
Power = density*n^2*D^5*CP;

% Downwash caused by propeller slipstream based on LabanOn-line Aircraft
% Aerodynamic Model Identification. PhD thesis, Proefschrift Technische
% Universiteit Delft, 1994.
e_p = (Forces(1)*sin(alpha)-Forces(3)*cos(alpha))/(density*V^2*Ap);
TC = Tc*pi/8;


end

== matlab function PropTest/Back propeller/MATLAB Function ==
  data: UVW input; TAS_prop output; PQR input; prop_pos input; alpha_prop output; beta_prop output; DCM_prop2b output
function [TAS_prop,alpha_prop,beta_prop,DCM_prop2b] = fcn(UVW,PQR,prop_pos)
%Initialize vectors
UVW = [UVW(1) UVW(2) UVW(3)];
% UVW = [-UVW(3) UVW(2) UVW(1)];%what it would like on that position, used
% b2prop axis matrix transformation instead
PQR = [PQR(1) PQR(2) PQR(3)];
prop_pos = [prop_pos(1) prop_pos(2) prop_pos(3)];

DCM_b2prop = [0 0 -1;
              0 1 0;
              1 0 0];
%UVW calculation v = v0 + w^r (rigid body)
WR_ba = cross(PQR,prop_pos);
UVW_prop = (DCM_b2prop*UVW')' + (DCM_b2prop*cross(PQR,prop_pos)')';

%outputs
TAS_prop = norm(UVW_prop);

if TAS_prop < 10
    alpha_prop = 0;
    beta_prop = 0;
else
    alpha_prop = atan(UVW_prop(3)/UVW_prop(1));
    beta_prop = asin(UVW_prop(2)/TAS_prop);
end
DCM_prop2b = [0 0 1;
        0 1 0;
        -1 0 0];
end
